simulink model "Rotor_model"  (R2022a)
settings: Solver=VariableStepAuto  StartTime=0.0  StopTime=30  MaxStep=0.01  RelTol=1e-3
settings Model: Creator=matm  LastModifiedBy=nikos
settings SolverCC: ShapePreserveControl=EnableAll  AlgebraicLoopSolver=TrustRegion  SolverResetMethod=Robust
settings DataIOCC: ReturnWorkspaceOutputs=off
settings DebuggingCC: UnconnectedInputMsg=warning  UnconnectedOutputMsg=warning  UnconnectedLineMsg=warning  SFMachineParentedDataDiag=warning  ArithmeticOperatorsInVariantConditions=warning
settings SFSimCC: SimUseLocalCustomCode=off  CustomCodeUndefinedFunction=UseInterfaceOnly
settings RTWCC: RTWUseLocalCustomCode=off  DLArmComputeVersion=19.05
settings CodeAppCC: StateflowObjectComments=on

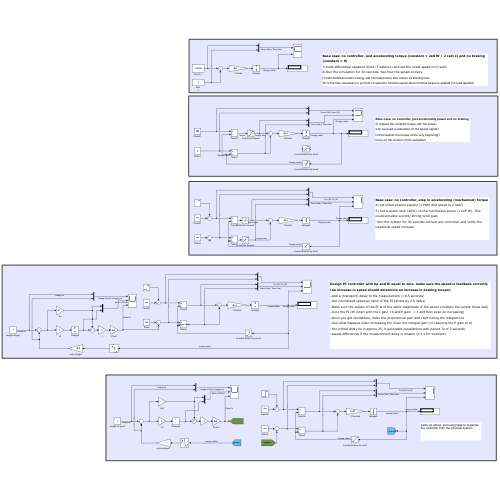
[thumbnail: Simulink's stored preview of the top-level diagram]
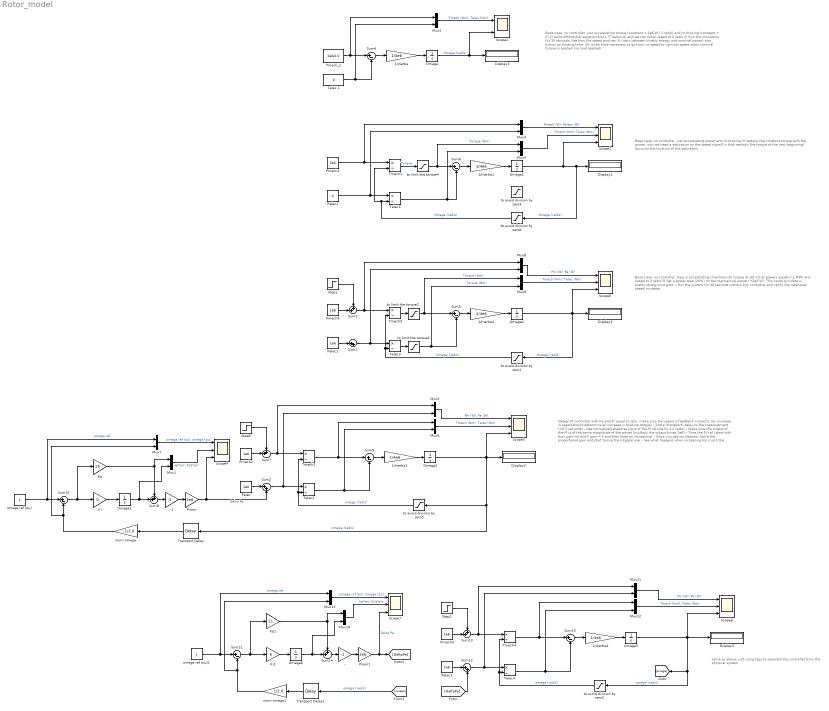
== system Rotor_model ==
  note: same as above, just using tags to separate the controller from the physical system
  note: Design PI controller with Kp and Ki equal to zero. make sure the speed is feedback correctly
      | (an increase in speed should determine an increase in braking torque)
      | – Add a (transport) delay to the measurement (=0.5 seconds)
      | – Use normalized speed as input of the PI (divide by 2.0 rad/s)
      | – Make sure the output of the PI is of the same magnitude of the power (multiply the output times 2e6)
      | – Tune the PI ctrl (start with the I gain =0 and P gain = 1 and then keep on increasing)
      | – Once you get oscillations, halve the proportional gain and start tuning the integral one
      | – See what happens when increasing too much the integral gain (or reducing the P gain to 0)
      | –the critical delay ku is approx 25, it generates osciallations with period Tu of 2 seconds
      | -assess differences if the measurement delay is smaller (0.1 s for example)
  note: Base case: no controller, just accelerating torque (constant = 2e6 W / 2 rad/s) and no braking (constant = 0)
      | 1) build differential equation block (T balance) and set the initial speed to 0 rad/s
      | 2) Run the simulation for 30 seconds. See how the speed evolves.
      | H (ratio between kinetic energy and nominal power) also known as starting time:
      | 2H is the time necessary to go from no speed to nominal speed when nominal torque is applied (no load applied)
  note: Base case: no controller, just accelerating power and no braking
      | 3) replace the constant torque with the power.
      | why we need a saturation on the speed signal?
      | is that realistic the torque at the very beginning?
      | focus on the location of the saturation
  note: Base case: no controller, step in accelerating (mechanical) torque
      | 4) set initial powers equally (1 MW) and speed to 2 rad/s
      | 5) Set a power step (20%) on the mechanical power (+2e5 W). This could simulate a pretty strong wind gust.
      | – Run the system for 30 seconds without any controller and verify the rotational speed increase
  - : Gain  Gain=-1
  -1 : Gain  Gain=-1
  1/Inertia{,1..4} (5 alike) : Gain  Gain=1/4e6
  Display{1..5} (5 alike) : Display
  Ki : Gain  Gain=0
  Ki1 : Gain  Gain=6
  Kp : Gain  Gain=25
  Kp1 : Gain  Gain=11
  Mux{1..13} (13 alike) : Mux  Inputs=2
  Omega{,1,3,6} (4 alike) : Integrator  ZeroCross=off
  Omega2 : Integrator  InitialCondition=2.0  ZeroCross=off
  Omega4 : Integrator  InitialCondition=2.0  ZeroCross=off
  Omega5 : Integrator  InitialCondition=2.0  ZeroCross=off
  Pelec : Constant  Value=1e6
  Pelec1 : Constant  Value=0
  Pelec2 : Constant  Value=1e6
  Pelec3 : Constant  Value=1e6
  Pmech1 : Constant  Value=2e6
  Pmech2 : Constant  Value=1e6
  Pmech3 : Constant  Value=1e6
  Pmech4 : Constant  Value=1e6
  Pnom : Gain  Gain=2e6
  Pnom1 : Gain  Gain=2e6
  Scope{1,3..7} (6 alike) : Scope  NumInputPorts=3
  Scope2 : Scope  NumInputPorts=2
  Step1 : Step  After=2e5  SampleTime=0
  Step2 : Step  After=2e5  SampleTime=0
  Step6 : Step  After=2e5  SampleTime=0
  Sum1 : Sum  Inputs=|++
  Sum{4..6,9..11,15} (7 alike) : Sum  Inputs=|+-
  Sum12 : Sum  Inputs=|++
  Sum{3,7..8,13..14} (5 alike) : Sum  Inputs=++|
  Sum2 : Sum  Inputs=|++
  Telec 1 : Constant  Value=0
  Telec{1..4} (4 alike) : Product  Inputs=*/
  Tmech{1..4} (4 alike) : Product  Inputs=*/
  "Tmech_1 " : Constant  Value=2e6/2.0
  Transport Delay : TransportDelay  DelayTime=0.5  InitialOutput=2
  Transport Delay1 : TransportDelay  DelayTime=0.5  InitialOutput=2
  norm omega : Gain  Gain=1/2.0
  norm omega1 : Gain  Gain=1/2.0
  omega ref (pu) : Constant
  omega ref (pu)1 : Constant
  to avoid division by zero{1..3,5..6} (5 alike) : Saturate  UpperLimit=inf  LowerLimit=0.001  ZeroCross=off
  to limit the torque2 : Saturate  UpperLimit=2e6/2  LowerLimit=0  ZeroCross=off
  to limit the torque3 : Saturate  UpperLimit=2e6/2  LowerLimit=0  ZeroCross=off
  to limit the torque4 : Saturate  UpperLimit=2e6/2  LowerLimit=0  ZeroCross=off
  wires:
  Omega/1 -> Scope2/2, Display3/1  "Omega (rad/s)"
  Sum4/1 -> 1/Inertia/1
  1/Inertia/1 -> Omega/1
  Telec 1/1 -> Mux2/2, Sum4/2
  Telec1/1 -> Mux4/2, Sum6/2
  Pmech1/1 -> Tmech1/1, Mux3/1
  Pelec1/1 -> Telec1/1, Mux3/2
  Mux3/1 -> Scope1/1  "Pmech (W); Pelect (W)"
  Mux4/1 -> Scope1/2  "Tmech (Nm); Telec (Nm)"
  1/Inertia1/1 -> Omega1/1
  Sum6/1 -> 1/Inertia1/1
  Sum9/1 -> 1/Inertia2/1
  1/Inertia2/1 -> Omega2/1
  Mux6/1 -> Scope3/2  "Tmech (Nm); Telec (Nm)"
  Mux5/1 -> Scope3/1  "Pm (W); Pe (W)"
  Pmech2/1 -> Sum7/2
  Omega2/1 -> Transport Delay/1, to avoid division by zero5/1, Scope3/3, Display2/1  "omega (rad/s)"
  Sum7/1 -> Mux5/1, Tmech2/1
  Tmech2/1 -> Sum9/1, Mux6/1
  Telec2/1 -> Sum9/2, Mux6/2
  Ki/1 -> Omega3/1
  Sum8/1 -> -1/1
  Kp/1 -> Mux1/1, Sum8/1
  Sum10/1 -> Kp/1, Ki/1
  omega ref (pu)/1 -> Mux7/1, Sum10/1  "omega ref"
  Mux2/1 -> Scope2/1  "Tmech (Nm); Telec (Nm)"
  Mux7/1 -> Scope4/1  "omega ref (pu); omega (pu)"
  Mux1/1 -> Scope4/2  "kp*err; Ki/s*err"
  Sum2/1 -> Mux5/2, Telec2/1
  -1/1 -> Pnom/1
  norm omega/1 -> Mux7/2, Sum10/2
  Pnom/1 -> Sum2/2, Scope4/3  "Delta Pe"
  Transport Delay/1 -> norm omega/1
  Step6/1 -> Sum7/1
  Pelec/1 -> Sum2/1
  "Tmech_1 "/1 -> Mux2/1, Sum4/1
  Tmech1/1 -> to limit the torque4/1  "Torque"
  Pelec2/1 -> Sum1/1
  Sum1/1 -> Telec3/1, Mux8/2
  Telec3/1 -> to limit the torque3/1
  Tmech3/1 -> to limit the torque2/1
  Sum3/1 -> Tmech3/1, Mux8/1
  Pmech3/1 -> Sum3/2
  Mux8/1 -> Scope5/1  "Pm (W); Pe (W)"
  Mux9/1 -> Scope5/2  "Tmech (Nm); Telec (Nm)"
  1/Inertia3/1 -> Omega4/1
  Sum5/1 -> 1/Inertia3/1
  Omega4/1 -> Display4/1, Scope5/3, to avoid division by zero1/1  "Omega (rad/s)"
  to avoid division by zero1/1 -> Telec3/2, Tmech3/2  "Omega (rad/s)"
  [omega] -> Transport Delay1/1  "omega (rad/s)"
  Omega6/1 -> Mux10/2, Sum14/2
  Pelec3/1 -> Sum12/1
  Step2/1 -> Sum13/1
  Transport Delay1/1 -> norm omega1/1
  Pnom1/1 -> [DeltaPe], Scope7/3  "Delta Pe"
  norm omega1/1 -> Sum11/2, Mux13/2
  -/1 -> Pnom1/1
  Sum12/1 -> Telec4/1, Mux11/2
  Mux10/1 -> Scope7/2  "kp*err; Ki/s*err"
  Mux13/1 -> Scope7/1  "omega ref (pu); omega (pu)"
  omega ref (pu)1/1 -> Sum11/1, Mux13/1  "omega ref"
  Sum11/1 -> Ki1/1, Kp1/1
  Kp1/1 -> Sum14/1, Mux10/1
  Sum14/1 -> -/1
  Ki1/1 -> Omega6/1
  Telec4/1 -> Mux12/2, Sum15/2
  Tmech4/1 -> Mux12/1, Sum15/1
  Sum13/1 -> Tmech4/1, Mux11/1
  Omega5/1 -> Display5/1, Scope6/3, to avoid division by zero2/1, [omega]  "omega (rad/s)"
  Pmech4/1 -> Sum13/2
  Mux11/1 -> Scope6/1  "Pm (W); Pe (W)"
  Mux12/1 -> Scope6/2  "Tmech (Nm); Telec (Nm)"
  1/Inertia4/1 -> Omega5/1
  Sum15/1 -> 1/Inertia4/1
  [DeltaPe] -> Sum12/2
  Omega3/1 -> Sum8/2, Mux1/2
  to avoid division by zero5/1 -> Tmech2/2, Telec2/2  "omega (rad/s)"
  to avoid division by zero2/1 -> Telec4/2, Tmech4/2  "omega (rad/s)"
  to limit the torque2/1 -> Mux9/1, Sum5/1  "Torque (Nm)"
  to limit the torque3/1 -> Mux9/2, Sum5/2  "Torque (Nm)"
  Omega1/1 -> to avoid division by zero6/1, Display1/1, Scope1/3  "Omega (rad/s)"
  to avoid division by zero6/1 -> Tmech1/2, Telec1/2  "Omega (rad/s)"
  to limit the torque4/1 -> Mux4/1, Sum6/1  "Torque (Nm)"
  Step1/1 -> Sum3/1
